simulink model "sine_wave"  (R2019b)
settings: Solver=VariableStepAuto  StartTime=0.0  StopTime=10.0  MaxStep=0.01  RelTol=1e-3
settings Model: Creator=dgander  LastModifiedBy=dgander

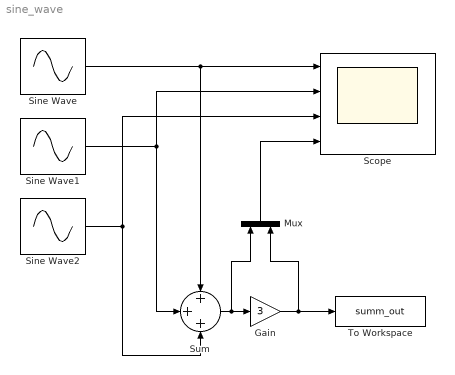
== system sine_wave ==
  Gain : Gain  Gain=3
  Mux : Mux  Inputs=2
  Scope : Scope  NumInputPorts=4
  Sine Wave : Sin  SampleTime=0
  Sine Wave1 : Sin  Frequency=5  SampleTime=0
  Sine Wave2 : Sin  Frequency=10  SampleTime=0
  Sum : Sum  Inputs=3
  To Workspace : ToWorkspace  VariableName=summ_out  SaveFormat=Timeseries  SampleTime=-1
  wires:
  Sine Wave/1 -> Sum/1, Scope/1
  Sine Wave1/1 -> Sum/2, Scope/2
  Sine Wave2/1 -> Sum/3, Scope/3
  Sum/1 -> Mux/1, Gain/1
  Gain/1 -> Mux/2, To Workspace/1
  Mux/1 -> Scope/4
